simulink model "feng_ct"  (R2016b)
settings: Solver=VariableStepAuto  StartTime=0.0  StopTime=5000  RelTol=1e-3  EnableMultiTasking=on
undefined symbols (not defined in the file or in its folder): fft_stages, output_len_bits, xengbits
undefined symbols (not defined in the file): input_bits, total_bits, total_bits2
libraries: xbsIndex_r4 x10571, casper_library_misc x48, casper_library_scopes x9, xps_library x2
(part 26 of 81)

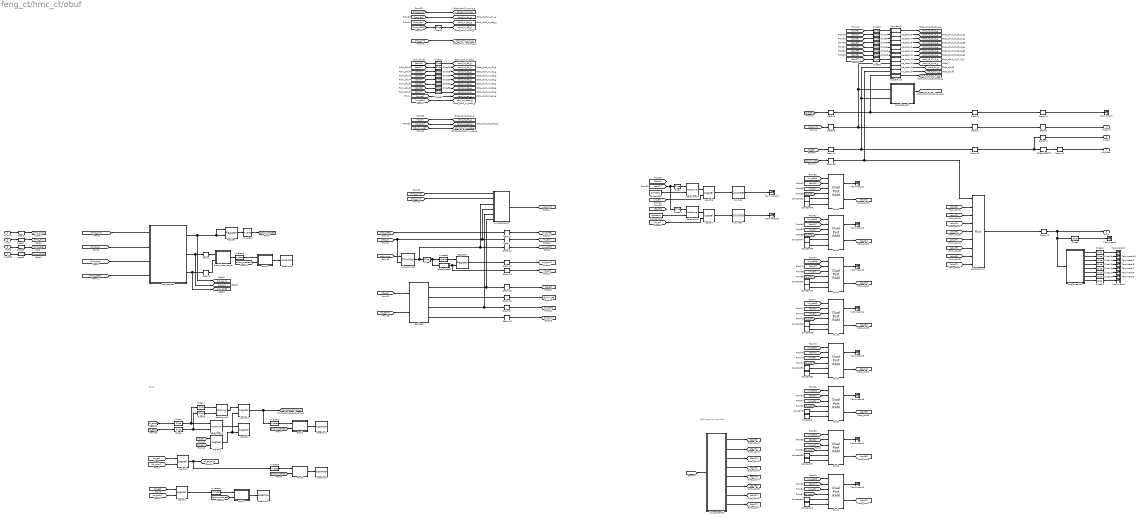
== system feng_ct/hmc_ct/obuf ==
  note: Errors
  note: Eight parallel channels.
  in_sync : Inport
  in_dv : Inport  Port=2
  in_tag : Inport  Port=3
  in_d256 : Inport  Port=4
  Assert : xbsIndex_r4/Assert  assert_type=on  type_source=Explicitly  gui_display_data_type=Boolean  arith_type=Boolean  n_bits=16  bin_pt=14  preci_type=Single  exp_width=8  frac_width=24  assert_rate=on  rate_source=Explicitly  period=1  output_port=on  block_type=assert
  Assert1 : xbsIndex_r4/Assert  assert_type=on  type_source=Explicitly  gui_display_data_type=Boolean  arith_type=Boolean  n_bits=16  bin_pt=14  preci_type=Single  exp_width=8  frac_width=24  assert_rate=on  rate_source=Explicitly  period=1  output_port=on  block_type=assert
  Assert2 : xbsIndex_r4/Assert  assert_type=on  type_source=Explicitly  gui_display_data_type=Fixed-point  arith_type=Unsigned  n_bits=9  bin_pt=0  preci_type=Single  exp_width=8  frac_width=24  assert_rate=on  rate_source=Explicitly  period=1  output_port=on  block_type=assert
  Assert3 : xbsIndex_r4/Assert  assert_type=on  type_source=Explicitly  gui_display_data_type=Fixed-point  arith_type=Unsigned  n_bits=256  bin_pt=0  preci_type=Single  exp_width=8  frac_width=24  assert_rate=on  rate_source=Explicitly  period=1  output_port=on  block_type=assert
  Assertion{1..3,5} (4 alike) : Assertion
  Constant{5,36,38,42,44,46,48,50} (8 alike) : xbsIndex_r4/Constant  const=0  gui_display_data_type=Fixed-point  arith_type=Unsigned  n_bits=256  bin_pt=0  preci_type=Single  exp_width=8  frac_width=24  explicit_period=on  period=1  equ=P=C  opselect=C  inp2=PCIN>>17  opr=+  inp1=P  carry=CIN  dbl_ovrd=off  block_type=constant
  Constant{6,37,41,43,45,47,49,51} (8 alike) : xbsIndex_r4/Constant  const=0  gui_display_data_type=Boolean  arith_type=Boolean  n_bits=256  bin_pt=0  preci_type=Single  exp_width=8  frac_width=24  explicit_period=on  period=1  equ=P=C  opselect=C  inp2=PCIN>>17  opr=+  inp1=P  carry=CIN  dbl_ovrd=off  block_type=constant
  Constant52 : xbsIndex_r4/Constant  const=14695  gui_display_data_type=Fixed-point  arith_type=Unsigned  n_bits=fft_stages-1  bin_pt=0  preci_type=Single  exp_width=8  frac_width=24  explicit_period=on  period=1  equ=P=C  opselect=C  inp2=PCIN>>17  opr=+  inp1=P  carry=CIN  dbl_ovrd=off  block_type=constant
  Constant53 : xbsIndex_r4/Constant  const=29031  gui_display_data_type=Fixed-point  arith_type=Unsigned  n_bits=fft_stages-1  bin_pt=0  preci_type=Single  exp_width=8  frac_width=24  explicit_period=on  period=1  equ=P=C  opselect=C  inp2=PCIN>>17  opr=+  inp1=P  carry=CIN  dbl_ovrd=off  block_type=constant
  Counter : xbsIndex_r4/Counter  cnt_type=Free Running  cnt_to=Inf  operation=Up  start_count=0  cnt_by_val=1  arith_type=Unsigned  n_bits=32  bin_pt=0  load_pin=off  rst=off  en=on  explicit_period=on  period=1  use_behavioral_HDL=off  implementation=Fabric  dbl_ovrd=off  block_type=counter
  Counter1 : xbsIndex_r4/Counter  cnt_type=Free Running  cnt_to=Inf  operation=Up  start_count=0  cnt_by_val=1  arith_type=Unsigned  n_bits=32  bin_pt=0  load_pin=off  rst=off  en=on  explicit_period=on  period=1  use_behavioral_HDL=off  implementation=Fabric  dbl_ovrd=off  block_type=counter
  Delay1 : xbsIndex_r4/Delay  rst=off  infoeditControl=Selection of Reset will increase slice count due to use of real FFs and instead of SRLs  en=off  latency=1  reg_retiming=off  dbl_ovrd=off  block_type=delay
      settings: infoedit=Hardware notes: A delay line is a chain, each link of which is an SRL16 or SRL32 followed by a flip-flop.
  Delay{4,7,10,12..18} (10 alike) : xbsIndex_r4/Delay  rst=off  infoeditControl=Selection of Reset will increase slice count due to use of real FFs and instead of SRLs  en=off  latency=2  reg_retiming=off  dbl_ovrd=off  block_type=delay
      settings: infoedit=Hardware notes: A delay line is a chain, each link of which is an SRL16 or SRL32 followed by a flip-flop.
  Delay{3,11,37,45} (4 alike) : xbsIndex_r4/Delay  rst=off  infoeditControl=Selection of Reset will increase slice count due to use of real FFs and instead of SRLs  en=off  latency=3  reg_retiming=off  dbl_ovrd=off  block_type=delay
      settings: infoedit=Hardware notes: A delay line is a chain, each link of which is an SRL16 or SRL32 followed by a flip-flop.
  Delay2 : xbsIndex_r4/Delay  rst=off  infoeditControl=Selection of Reset will increase slice count due to use of real FFs and instead of SRLs  en=off  latency=1  reg_retiming=off  dbl_ovrd=off  block_type=delay
      settings: infoedit=Hardware notes: A delay line is a chain, each link of which is an SRL16 or SRL32 followed by a flip-flop.
  Delay{6,8,36,42} (4 alike) : xbsIndex_r4/Delay  rst=off  infoeditControl=Selection of Reset will increase slice count due to use of real FFs and instead of SRLs  en=off  latency=pkt_buffer_latency  reg_retiming=off  dbl_ovrd=off  block_type=delay
      settings: infoedit=Hardware notes: A delay line is a chain, each link of which is an SRL16 or SRL32 followed by a flip-flop.
  Delay43 : xbsIndex_r4/Delay  rst=off  infoeditControl=Selection of Reset will increase slice count due to use of real FFs and instead of SRLs  en=off  latency=omux_latency  reg_retiming=off  dbl_ovrd=off  block_type=delay
      settings: infoedit=Hardware notes: A delay line is a chain, each link of which is an SRL16 or SRL32 followed by a flip-flop.
  Delay5 : xbsIndex_r4/Delay  rst=off  infoeditControl=Selection of Reset will increase slice count due to use of real FFs and instead of SRLs  en=off  latency=omux_latency  reg_retiming=off  dbl_ovrd=off  block_type=delay
      settings: infoedit=Hardware notes: A delay line is a chain, each link of which is an SRL16 or SRL32 followed by a flip-flop.
  Delay9 : xbsIndex_r4/Delay  rst=off  infoeditControl=Selection of Reset will increase slice count due to use of real FFs and instead of SRLs  en=off  latency=omux_latency  reg_retiming=off  dbl_ovrd=off  block_type=delay
      settings: infoedit=Hardware notes: A delay line is a chain, each link of which is an SRL16 or SRL32 followed by a flip-flop.
  Inverter{1..6} (6 alike) : xbsIndex_r4/Inverter  en=off  latency=0  dbl_ovrd=off  block_type=inv
  Logical1 : xbsIndex_r4/Logical  logical_function=AND  inputs=2  en=off  latency=1  precision=Full  arith_type=Unsigned  n_bits=16  bin_pt=0  align_bp=on  dbl_ovrd=off  block_type=logical
  Logical{2..3,6..7,9} (5 alike) : xbsIndex_r4/Logical  logical_function=AND  inputs=2  en=off  latency=0  precision=Full  arith_type=Unsigned  n_bits=16  bin_pt=0  align_bp=on  dbl_ovrd=off  block_type=logical
  Logical4 : xbsIndex_r4/Logical  logical_function=AND  inputs=2  en=off  latency=1  precision=Full  arith_type=Unsigned  n_bits=16  bin_pt=0  align_bp=on  dbl_ovrd=off  block_type=logical
  Register : xbsIndex_r4/Register  init=0  rst=off  en=on  dbl_ovrd=off  block_type=register
  Register1 : xbsIndex_r4/Register  init=0  rst=off  en=on  dbl_ovrd=off  block_type=register
  Relational{2..4,6} (4 alike) : xbsIndex_r4/Relational  mode=a=b  op_type=Bool  en=off  latency=0  dbl_ovrd=off  block_type=relational
  Slice : xbsIndex_r4/Slice  nbits=1  boolean_output=on  mode=Upper Bit Location + Width  bit1=0  base1=MSB of Input  bit0=0  base0=LSB of Input  dbl_ovrd=off  block_type=slice
  Slice1 : xbsIndex_r4/Slice  nbits=1  boolean_output=off  mode=Two Bit Locations  bit1=0  base1=MSB of Input  bit0=0  base0=LSB of Input  dbl_ovrd=off  block_type=slice
  Slice{10..16,20} (8 alike) : xbsIndex_r4/Slice  nbits=9  boolean_output=off  mode=Lower Bit Location + Width  bit1=0  base1=MSB of Input  bit0=0  base0=LSB of Input  dbl_ovrd=off  block_type=slice
  Slice17 : xbsIndex_r4/Slice  nbits=1  boolean_output=off  mode=Two Bit Locations  bit1=0  base1=MSB of Input  bit0=5  base0=LSB of Input  dbl_ovrd=off  block_type=slice
  Slice18 : xbsIndex_r4/Slice  nbits=1  boolean_output=off  mode=Two Bit Locations  bit1=0  base1=MSB of Input  bit0=5  base0=LSB of Input  dbl_ovrd=off  block_type=slice
  Slice19 : xbsIndex_r4/Slice  nbits=15  boolean_output=off  mode=Upper Bit Location + Width  bit1=-1  base1=MSB of Input  bit0=0  base0=LSB of Input  dbl_ovrd=off  block_type=slice
  Slice{6..9,22..34} (17 alike) : xbsIndex_r4/Slice  nbits=fft_stages-1  boolean_output=off  mode=Upper Bit Location + Width  bit1=-1*(16-(fft_stages-1))  base1=MSB of Input  bit0=0  base0=LSB of Input  dbl_ovrd=off  block_type=slice
  Slice3 : xbsIndex_r4/Slice  nbits=15  boolean_output=off  mode=Upper Bit Location + Width  bit1=-1  base1=MSB of Input  bit0=0  base0=LSB of Input  dbl_ovrd=off  block_type=slice
  Slice4 : xbsIndex_r4/Slice  nbits=16  boolean_output=off  mode=Upper Bit Location + Width  bit1=0  base1=MSB of Input  bit0=0  base0=LSB of Input  dbl_ovrd=off  block_type=slice
  Slice5 : xbsIndex_r4/Slice  nbits=1  boolean_output=off  mode=Two Bit Locations  bit1=0  base1=MSB of Input  bit0=3  base0=LSB of Input  dbl_ovrd=off  block_type=slice
  Terminator{1,3..19,22..23} (20 alike) : Terminator
  bus_expand1 : Subsystem  AncestorBlock=casper_library_flow_control/bus_expand  mask(bus_expand){mode=divisions of equal size, outputNum=8, outputWidth=32, outputBinaryPt=0, outputArithmeticType=0, show_format=on, outputToWorkspace=off, variablePrefix=out, outputToModelAsWell=on}
      mask prompts: outputNum "Number of outputs:"; outputWidth "Output width:"; outputBinaryPt "Output binary point position:"; outputArithmeticType "Output arithmetic type (ufix=0, fix=1, bool=2):"; show_format "Print format string?"; outputToWorkspace "Output to workspace?"; variablePrefix "Variable name prefix:"; outputToModelAsWell "Output to model as well?"
      mask help:
      | Expands a 'bus' made using a bus_create or Xilinx
      | concat block.
      | The input will be divided into the specified number
      | of outputs with the specified arithmetic types.
      | Divisions are made from most significant bit.
      mask init: same as feng_ct/bus_expand1
      settings: AttributesFormatString=8 outputs: uf32.0,uf32.0,uf32.0,uf32.0,uf32.0,uf32.0,uf32.0,uf32.0,
      mask TypeOptions mode: divisions of equal size | divisions of arbitrary size
      mask Callback mode: bus_expand_callback();
      mask Callback outputWidth: bus_expand_callback();
      mask Callback outputToWorkspace: bus_expand_callback();
  bus_expand3 : Subsystem  AncestorBlock=casper_library_flow_control/bus_expand  mask(bus_expand){mode=divisions of equal size, outputNum=8, outputWidth=32, outputBinaryPt=0, outputArithmeticType=0, show_format=off, outputToWorkspace=off, variablePrefix=out, outputToModelAsWell=on}
      mask prompts: outputNum "Number of outputs:"; outputWidth "Output width:"; outputBinaryPt "Output binary point position:"; outputArithmeticType "Output arithmetic type (ufix=0, fix=1, bool=2):"; show_format "Print format string?"; outputToWorkspace "Output to workspace?"; variablePrefix "Variable name prefix:"; outputToModelAsWell "Output to model as well?"
      mask help:
      | Expands a 'bus' made using a bus_create or Xilinx
      | concat block.
      | The input will be divided into the specified number
      | of outputs with the specified arithmetic types.
      | Divisions are made from most significant bit.
      mask init: same as feng_ct/bus_expand1
      settings: AttributesFormatString=8 outputs
      mask TypeOptions mode: divisions of equal size | divisions of arbitrary size
      mask Callback mode: bus_expand_callback();
      mask Callback outputWidth: bus_expand_callback();
      mask Callback outputToWorkspace: bus_expand_callback();
  check_data_length : Subsystem
  edge_detect : Subsystem  AncestorBlock=casper_library_misc/edge_detect  mask(edge_detect){edge=Both, polarity=Active High, x_in=[0 0.08 0.08 0.16 0.16 0.24 0.24 0.32 0.32 0.4], y_in=[-1 -1  1  1  1  1  1  1  1  1], x_out=[0.6 0.68 0.68 0.76 0.76 0.84 0.84 0.92 0.92 1], y_out=[-1 -1  1  1 -1 -1 -1 -1 -1 -1]}
      mask prompts: edge "Edge Type"; polarity "Output Polarity"; x_in "Input X Positions"; y_in "Input Y Positions"; x_out "Output X Positions"; y_out "Output Y Positions"
      mask help: Output is active for one-cycle after each edge of the specified type (i.e. rising, falling or both).
      mask init: same as feng_ct/edge_detect1
      settings: AttributesFormatString=|
      | both edges
      | active high
      mask Help: Output is active for one-cycle after each edge of the specified type (i.e. rising, falling, or both).  Latency is zero.
      mask TypeOptions edge: Rising | Falling | Both
      mask TypeOptions polarity: Active High | Active Low
      mask Display:
      | plot(x_in_num,0.5+y_in_num*0.2);
      | plot(x_out_num,0.5+y_out_num*0.2);
  edge_detect1 : casper_library_misc/edge_detect  edge=Rising  polarity=Active High  x_in=[0 0.08 0.08 0.16 0.16 0.24 0.24 0.32 0.32 0.4]  y_in="[-1 -1  1  1  1  1  1  1  1  1]"  x_out=[0.6 0.68 0.68 0.76 0.76 0.84 0.84 0.92 0.92 1]  y_out="[-1 -1  1  1 -1 -1 -1 -1 -1 -1]"
  error1 : Subsystem
  error2 : Subsystem
  error3 : Subsystem
  error4 : Subsystem
  gen_freq_calc : Subsystem  mask{pkt_len_bits=5, lat=3}
      mask prompts: pkt_len_bits "Packet length bits"; lat "Latency"
      mask init:
      | display_string = sprintf('latency=%i', 7 * lat);
      | set_param(gcb, 'AttributesFormatString', display_string);
      settings: AttributesFormatString=latency=21
  obuf0 : xbsIndex_r4/Dual Port RAM  depth=2^(output_len_bits + 2)  initVector=ones(1, 2^(output_len_bits + 2))  distributed_mem=Block RAM  init_a=0  init_b=0  rst_a=off  rst_b=off  en_a=off  en_b=off  latency=pkt_buffer_latency  write_mode_A=Read Before Write  write_mode_B=Read Before Write  optimize=Area  dbl_ovrd=off  block_type=dpram
  obuf{1..7} (7 alike) : xbsIndex_r4/Dual Port RAM  depth=2^(output_len_bits + 2)  initVector=zeros(1, 2^(output_len_bits + 2))  distributed_mem=Block RAM  init_a=0  init_b=0  rst_a=off  rst_b=off  en_a=off  en_b=off  latency=pkt_buffer_latency  write_mode_A=Read Before Write  write_mode_B=Read Before Write  optimize=Area  dbl_ovrd=off  block_type=dpram
  pkt_data_mux : xbsIndex_r4/Mux  inputs=8  en=off  latency=omux_latency  precision=Full  arith_type=Unsigned  n_bits=16  bin_pt=14  quantization=Truncate  overflow=Wrap  dbl_ovrd=off  block_type=mux
  read_gen : Subsystem
  sync_generator : Subsystem
  tag_reorder : Subsystem
  we_delay1 : Subsystem  AncestorBlock=casper_library_delays/pipeline  mask(pipeline){latency=21}
      mask help:
      | An explicitly laid-out delay line to avoid mapping to SRL16s
      | for use in pipelining to help achieve timing closure.
      mask init:
      | pipeline_init(gcb,'latency',latency);
      settings: AttributesFormatString=Latency = %<latency>
      mask Display:
      | port_label('input', 1, 'd');
      | port_label('output', 1, 'q');
      | disp(['Z^-', num2str(latency)]);
  we_delay10 : Subsystem  AncestorBlock=casper_library_delays/pipeline  mask(pipeline){latency=21}
      mask help:
      | An explicitly laid-out delay line to avoid mapping to SRL16s
      | for use in pipelining to help achieve timing closure.
      mask init:
      | pipeline_init(gcb,'latency',latency);
      settings: AttributesFormatString=Latency = %<latency>
      mask Display:
      | port_label('input', 1, 'd');
      | port_label('output', 1, 'q');
      | disp(['Z^-', num2str(latency)]);
  we_delay11 : Subsystem  AncestorBlock=casper_library_delays/pipeline  mask(pipeline){latency=21}
      mask help:
      | An explicitly laid-out delay line to avoid mapping to SRL16s
      | for use in pipelining to help achieve timing closure.
      mask init:
      | pipeline_init(gcb,'latency',latency);
      settings: AttributesFormatString=Latency = %<latency>
      mask Display:
      | port_label('input', 1, 'd');
      | port_label('output', 1, 'q');
      | disp(['Z^-', num2str(latency)]);
  we_delay12 : Subsystem  AncestorBlock=casper_library_delays/pipeline  mask(pipeline){latency=21}
      mask help:
      | An explicitly laid-out delay line to avoid mapping to SRL16s
      | for use in pipelining to help achieve timing closure.
      mask init:
      | pipeline_init(gcb,'latency',latency);
      settings: AttributesFormatString=Latency = %<latency>
      mask Display:
      | port_label('input', 1, 'd');
      | port_label('output', 1, 'q');
      | disp(['Z^-', num2str(latency)]);
  we_delay13 : Subsystem  AncestorBlock=casper_library_delays/pipeline  mask(pipeline){latency=21}
      mask help:
      | An explicitly laid-out delay line to avoid mapping to SRL16s
      | for use in pipelining to help achieve timing closure.
      mask init:
      | pipeline_init(gcb,'latency',latency);
      settings: AttributesFormatString=Latency = %<latency>
      mask Display:
      | port_label('input', 1, 'd');
      | port_label('output', 1, 'q');
      | disp(['Z^-', num2str(latency)]);
  we_delay2 : Subsystem  AncestorBlock=casper_library_delays/pipeline  mask(pipeline){latency=21}
      mask help:
      | An explicitly laid-out delay line to avoid mapping to SRL16s
      | for use in pipelining to help achieve timing closure.
      mask init:
      | pipeline_init(gcb,'latency',latency);
      settings: AttributesFormatString=Latency = %<latency>
      mask Display:
      | port_label('input', 1, 'd');
      | port_label('output', 1, 'q');
      | disp(['Z^-', num2str(latency)]);
  we_delay3 : Subsystem  AncestorBlock=casper_library_delays/pipeline  mask(pipeline){latency=21}
      mask help:
      | An explicitly laid-out delay line to avoid mapping to SRL16s
      | for use in pipelining to help achieve timing closure.
      mask init:
      | pipeline_init(gcb,'latency',latency);
      settings: AttributesFormatString=Latency = %<latency>
      mask Display:
      | port_label('input', 1, 'd');
      | port_label('output', 1, 'q');
      | disp(['Z^-', num2str(latency)]);
  we_delay5 : Subsystem  AncestorBlock=casper_library_delays/pipeline  mask(pipeline){latency=21}
      mask help:
      | An explicitly laid-out delay line to avoid mapping to SRL16s
      | for use in pipelining to help achieve timing closure.
      mask init:
      | pipeline_init(gcb,'latency',latency);
      settings: AttributesFormatString=Latency = %<latency>
      mask Display:
      | port_label('input', 1, 'd');
      | port_label('output', 1, 'q');
      | disp(['Z^-', num2str(latency)]);
  we_delay6 : Subsystem  AncestorBlock=casper_library_delays/pipeline  mask(pipeline){latency=21}
      mask help:
      | An explicitly laid-out delay line to avoid mapping to SRL16s
      | for use in pipelining to help achieve timing closure.
      mask init:
      | pipeline_init(gcb,'latency',latency);
      settings: AttributesFormatString=Latency = %<latency>
      mask Display:
      | port_label('input', 1, 'd');
      | port_label('output', 1, 'q');
      | disp(['Z^-', num2str(latency)]);
  we_delay7 : Subsystem  AncestorBlock=casper_library_delays/pipeline  mask(pipeline){latency=21}
      mask help:
      | An explicitly laid-out delay line to avoid mapping to SRL16s
      | for use in pipelining to help achieve timing closure.
      mask init:
      | pipeline_init(gcb,'latency',latency);
      settings: AttributesFormatString=Latency = %<latency>
      mask Display:
      | port_label('input', 1, 'd');
      | port_label('output', 1, 'q');
      | disp(['Z^-', num2str(latency)]);
  we_delay8 : Subsystem  AncestorBlock=casper_library_delays/pipeline  mask(pipeline){latency=21}
      mask help:
      | An explicitly laid-out delay line to avoid mapping to SRL16s
      | for use in pipelining to help achieve timing closure.
      mask init:
      | pipeline_init(gcb,'latency',latency);
      settings: AttributesFormatString=Latency = %<latency>
      mask Display:
      | port_label('input', 1, 'd');
      | port_label('output', 1, 'q');
      | disp(['Z^-', num2str(latency)]);
  we_delay9 : Subsystem  AncestorBlock=casper_library_delays/pipeline  mask(pipeline){latency=21}
      mask help:
      | An explicitly laid-out delay line to avoid mapping to SRL16s
      | for use in pipelining to help achieve timing closure.
      mask init:
      | pipeline_init(gcb,'latency',latency);
      settings: AttributesFormatString=Latency = %<latency>
      mask Display:
      | port_label('input', 1, 'd');
      | port_label('output', 1, 'q');
      | disp(['Z^-', num2str(latency)]);
  write_counter : xbsIndex_r4/Counter  cnt_type=Free Running  cnt_to=Inf  operation=Up  start_count=0  cnt_by_val=1  arith_type=Unsigned  n_bits=10  bin_pt=0  load_pin=off  rst=on  en=on  explicit_period=on  period=1  use_behavioral_HDL=off  implementation=Fabric  dbl_ovrd=off  block_type=counter
  out_sync : Outport
  out_dv : Outport  Port=2
  out_d : Outport  Port=3
  pkt_start : Outport  Port=4
  tag scope: obuf_ct_addr_err_g=global, obuf_dv_g=global, obuf_in_d0_g=global, obuf_in_dv_g=global, obuf_in_sync_g=global, obuf_in_tag_g=global, obuf_mux_g=global, obuf_premux_freq_ctr_g=global, obuf_proc_sync_g=global, obuf_rd_addr_g=global, obuf_rd_addr_out_g=global, obuf_rd_d0_0_g=global, obuf_rd_d1_0_g=global, obuf_rd_d2_0_g=global, obuf_rd_d3_0_g=global, obuf_rd_d4_0_g=global, obuf_rd_d5_0_g=global, obuf_rd_d6_0_g=global, obuf_rd_d7_0_g=global, obuf_rd_en_g=global, obuf_rd_mux_sel_g=global, obuf_rd_sync_g=global, obuf_wr_addr_g=global, obuf_wr_d0_g=global, obuf_wr_d1_g=global, obuf_wr_d2_g=global, obuf_wr_d3_g=global, obuf_wr_d4_g=global, obuf_wr_d5_g=global, obuf_wr_d6_g=global, obuf_wr_d7_g=global, obuf_wr_en_g=global, proc_d256=global, proc_dv=global, proc_sync=global, rd_go_err_g=global
  wires:
  in_dv/1 -> Assert1/1  "IN_dv"
  in_tag/1 -> Assert2/1
  in_sync/1 -> Assert/1  "IN_sync"
  [rd_en] -> Logical9/1
  [wr_en] -> Logical9/2
  Logical9/1 -> Logical3/2, Logical2/2
  [rd_go] -> Logical4/1
  [rd_busy] -> Logical4/2
  Logical4/1 -> Inverter5/1, [rd_go_err_g]  "GO_ERROR"
  in_d256/1 -> Assert3/1
  [wr_addr] -> Slice5/1
  [rd_addr] -> Slice1/1
  Slice5/1 -> Slice17/1, Relational2/1  "WR_ADDR7"
  Slice1/1 -> Slice18/1, Relational2/2  "RD_ADDR7"
  Relational2/1 -> Logical2/1
  Logical3/1 -> Inverter2/1, [obuf_ct_addr_err_g]  "BANK_CLASH"
  Slice18/1 -> Relational3/2  "RD_ADDR2"
  Slice17/1 -> Relational3/1  "WR_ADDR2"
  Relational3/1 -> Logical3/1
  [hmc_d256] -> tag_reorder/4(in_d256)
  [hmc_tag] -> tag_reorder/3(in_tag)
  [hmc_dv] -> tag_reorder/2(in_dv)
  [hmc_sync] -> tag_reorder/1(in_sync)
  check_data_length/1(error) -> Inverter6/1
  tag_reorder/3(out_d256) -> [proc_d256], Delay2/1
  tag_reorder/2(out_dv) -> [proc_dv], Delay1/1
  Inverter6/1 -> error4/1(err)
  error4/1(err_out) -> Assertion5/1
  tag_reorder/1(out_sync) -> [proc_sync], Register/2, Register/1  "PROC_sync"
  Register/1 -> Inverter1/1
  Inverter1/1 -> [errors_masked]
  [errors_masked] -> error4/2(armed)
  Delay1/1 -> check_data_length/1(dv)
  Delay2/1 -> check_data_length/2(data)
  [rd_go] -> Logical1/1
  [rd_busy] -> Logical1/2
  Logical1/1 -> Inverter4/1  "RD_BUSY_CLASH"
  Inverter4/1 -> error2/1(err)
  error2/1(err_out) -> Assertion2/1
  [errors_masked] -> error2/2(armed)
  [wr_en] -> [obuf_wr_en_g]
  [wr_addr] -> [obuf_wr_addr_g]
  [rd_addr] -> [obuf_rd_addr_g]
  [rd_mux_sel] -> [obuf_rd_mux_sel_g]
  [rd_en] -> [obuf_rd_en_g]
  [hmc_sync] -> [obuf_in_sync_g]
  [hmc_d256] -> Slice22/1
  Slice22/1 -> [obuf_in_d0_g]
  [hmc_dv] -> [obuf_in_dv_g]
  [hmc_tag] -> [obuf_in_tag_g]
  [dbuf0] -> Slice27/1
  Slice27/1 -> [obuf_wr_d0_g]
  [dbuf1] -> Slice28/1
  [dbuf2] -> Slice29/1
  [dbuf3] -> Slice30/1
  [dbuf4] -> Slice31/1
  [dbuf5] -> Slice32/1
  [dbuf6] -> Slice33/1
  [dbuf7] -> Slice34/1
  Slice28/1 -> [obuf_wr_d1_g]
  Slice29/1 -> [obuf_wr_d2_g]
  Slice30/1 -> [obuf_wr_d3_g]
  Slice31/1 -> [obuf_wr_d4_g]
  Slice32/1 -> [obuf_wr_d5_g]
  Slice33/1 -> [obuf_wr_d6_g]
  Slice34/1 -> [obuf_wr_d7_g]
  [dbuf5] -> obuf5/2
  [wr_addr] -> obuf5/1
  [wr_en] -> obuf5/3
  [rd_addr] -> obuf5/4
  Constant5/1 -> obuf5/5
  Constant6/1 -> obuf5/6
  bus_expand1/8(lsb_out1) -> Slice20/1
  bus_expand1/7(out2) -> Slice10/1
  bus_expand1/6(out3) -> Slice11/1
  bus_expand1/5(out4) -> Slice12/1
  Slice12/1 -> Terminator7/1  "tag3"
  Slice11/1 -> Terminator6/1  "tag2"
  Slice10/1 -> Terminator5/1  "tag1"
  Slice20/1 -> Terminator4/1  "tag0"
  bus_expand1/1(msb_out8) -> Slice16/1
  bus_expand1/2(out7) -> Slice15/1
  bus_expand1/3(out6) -> Slice14/1
  Slice16/1 -> Terminator17/1
  Slice15/1 -> Terminator16/1
  Slice14/1 -> Terminator9/1
  Slice13/1 -> Terminator8/1
  bus_expand1/4(out5) -> Slice13/1
  obuf5/2 -> [obuf5]
  obuf5/1 -> Terminator18/1
  [dbuf6] -> obuf6/2
  [wr_addr] -> obuf6/1
  [wr_en] -> obuf6/3
  [rd_addr] -> obuf6/4
  Constant36/1 -> obuf6/5
  Constant37/1 -> obuf6/6
  obuf6/2 -> [obuf6]
  obuf6/1 -> Terminator19/1
  [dbuf7] -> obuf7/2
  [wr_addr] -> obuf7/1
  [wr_en] -> obuf7/3
  [rd_addr] -> obuf7/4
  Constant38/1 -> obuf7/5
  Constant41/1 -> obuf7/6
  obuf7/2 -> [obuf7]
  obuf7/1 -> Terminator10/1
  [dbuf0] -> obuf0/2
  [wr_addr] -> obuf0/1
  [wr_en] -> obuf0/3
  [rd_addr] -> obuf0/4
  Constant42/1 -> obuf0/5
  Constant43/1 -> obuf0/6
  obuf0/2 -> [obuf0]
  obuf0/1 -> Terminator11/1
  [dbuf1] -> obuf1/2
  [wr_addr] -> obuf1/1
  [wr_en] -> obuf1/3
  [rd_addr] -> obuf1/4
  Constant44/1 -> obuf1/5
  Constant45/1 -> obuf1/6
  obuf1/2 -> [obuf1]
  obuf1/1 -> Terminator12/1
  [dbuf2] -> obuf2/2
  [wr_addr] -> obuf2/1
  [wr_en] -> obuf2/3
  [rd_addr] -> obuf2/4
  Constant46/1 -> obuf2/5
  Constant47/1 -> obuf2/6
  obuf2/2 -> [obuf2]
  obuf2/1 -> Terminator13/1
  [dbuf3] -> obuf3/2
  [wr_addr] -> obuf3/1
  [wr_en] -> obuf3/3
  [rd_addr] -> obuf3/4
  Constant48/1 -> obuf3/5
  Constant49/1 -> obuf3/6
  obuf3/2 -> [obuf3]
  obuf3/1 -> Terminator14/1
  [dbuf4] -> obuf4/2
  [wr_addr] -> obuf4/1
  [wr_en] -> obuf4/3
  [rd_addr] -> obuf4/4
  Constant50/1 -> obuf4/5
  Constant51/1 -> obuf4/6
  obuf4/2 -> [obuf4]
  obuf4/1 -> Terminator15/1
  [rd_mux_sel] -> Delay36/1
  [obuf4] -> pkt_data_mux/6
  [obuf6] -> pkt_data_mux/8
  [obuf5] -> pkt_data_mux/7
  [obuf7] -> pkt_data_mux/9
  [obuf3] -> pkt_data_mux/5
  [obuf2] -> pkt_data_mux/4
  [obuf0] -> pkt_data_mux/2
  [obuf1] -> pkt_data_mux/3
  [rd_en] -> Delay42/1
  Delay45/1 -> out_d/1, Slice4/1, bus_expand1/1(bus_in)
  Delay37/1 -> out_dv/1  "out_dv"
  pkt_data_mux/1 -> Delay45/1
  [wr_d256] -> bus_expand3/1(bus_in)
  bus_expand3/1(msb_out8) -> [dbuf0]
  bus_expand3/2(out7) -> [dbuf1]
  bus_expand3/3(out6) -> [dbuf2]
  bus_expand3/4(out5) -> [dbuf3]
  bus_expand3/5(out4) -> [dbuf4]
  bus_expand3/6(out3) -> [dbuf5]
  bus_expand3/7(out2) -> [dbuf6]  "DATA_TAG"
  bus_expand3/8(lsb_out1) -> [dbuf7]
  Slice4/1 -> Terminator3/1  "out_freq"
  Delay36/1 -> pkt_data_mux/1, we_delay3/1(d)  "obuf_mux"
  Delay42/1 -> gen_freq_calc/2(dv), we_delay2/1(d), Delay43/1  "obuf_en"
  [obuf0] -> Slice23/1
  Slice23/1 -> we_delay5/1(d)  "obuf0"
  [obuf7] -> Slice26/1
  Slice26/1 -> we_delay12/1(d)
  [obuf1] -> Slice7/1
  Slice7/1 -> we_delay6/1(d)
  [obuf2] -> Slice8/1
  Slice8/1 -> we_delay7/1(d)
  [obuf3] -> Slice9/1
  Slice9/1 -> we_delay8/1(d)
  [obuf4] -> Slice6/1
  Slice6/1 -> we_delay9/1(d)
  [obuf5] -> Slice24/1
  Slice24/1 -> we_delay10/1(d)
  [obuf6] -> Slice25/1
  Slice25/1 -> we_delay11/1(d)
  we_delay2/1(q) -> [obuf_dv_g]
  we_delay3/1(q) -> [obuf_mux_g]
  we_delay13/1(q) -> [obuf_rd_addr_out_g]
  we_delay5/1(q) -> [obuf_rd_d0_0_g]
  we_delay6/1(q) -> [obuf_rd_d1_0_g]
  we_delay8/1(q) -> [obuf_rd_d3_0_g]
  we_delay7/1(q) -> [obuf_rd_d2_0_g]
  we_delay12/1(q) -> [obuf_rd_d7_0_g]
  we_delay11/1(q) -> [obuf_rd_d6_0_g]
  we_delay9/1(q) -> [obuf_rd_d4_0_g]
  we_delay10/1(q) -> [obuf_rd_d5_0_g]
  Delay5/1 -> Delay3/1  "out_sync"
  [rd_addr] -> Delay8/1
  Delay8/1 -> we_delay13/1(d), Delay9/1
  Delay11/1 -> Terminator1/1  "out_addr"
  Delay9/1 -> Delay11/1
  edge_detect1/1 -> Delay10/1
  Delay43/1 -> Delay37/1, edge_detect1/1
  Delay10/1 -> pkt_start/1  "out_pkt_start"
  we_delay1/1(q) -> [obuf_rd_sync_g]
  Delay6/1 -> gen_freq_calc/1(sync), we_delay1/1(d), Delay5/1
  [dbuf7] -> Slice19/1, Slice3/1
  Constant52/1 -> Relational4/2
  Relational4/1 -> Logical6/1
  [wr_en] -> Logical6/2
  Logical6/1 -> Counter/1  "WR_14695"
  Counter/1 -> Terminator22/1  "20504"
  Constant53/1 -> Relational6/2
  Relational6/1 -> Logical7/1
  [wr_en] -> Logical7/2
  Logical7/1 -> Counter1/1  "WR_29031"
  Counter1/1 -> Terminator23/1  "22552"
  Slice3/1 -> Relational4/1
  Slice19/1 -> Relational6/1
  Assert/1 -> [hmc_sync]
  Assert1/1 -> [hmc_dv]
  Assert2/1 -> [hmc_tag]
  Assert3/1 -> [hmc_d256]
  Inverter2/1 -> error1/1(err)
  error1/1(err_out) -> Assertion1/1
  [errors_masked] -> error1/2(armed)
  Inverter5/1 -> error3/1(err)
  error3/1(err_out) -> Assertion3/1
  [errors_masked] -> error3/2(armed)
  Delay3/1 -> out_sync/1
  gen_freq_calc/2(freq) -> [obuf_premux_freq_ctr_g]
  [proc_sync] -> write_counter/1
  [proc_dv] -> write_counter/2, sync_generator/4(wr_en), Delay7/1
  write_counter/1 -> sync_generator/3(wr_addr), Delay12/1, Slice/1  "WR_addr"
  Slice/1 -> Inverter3/1, edge_detect/1(in)  "WR_bank"
  Inverter3/1 -> Register1/1
  edge_detect/1(out) -> Delay14/1, Register1/2  "RD_go"
  Register1/1 -> Delay13/1
  read_gen/2(mux_sel) -> Delay16/1
  read_gen/1(dv) -> sync_generator/6(rd_en), Delay15/1
  read_gen/3(addr) -> Delay17/1, sync_generator/5(rd_addr)
  read_gen/4(rd_busy) -> Delay18/1
  [rd_bank] -> read_gen/2(bank)
  [rd_go] -> read_gen/1(go)
  [proc_d256] -> Delay4/1
  [proc_sync] -> sync_generator/2(proc_sync)  "PROC_sync"
  [hmc_sync] -> sync_generator/1(hmc_sync)  "HMC_sync"
  Delay4/1 -> [wr_d256]  "WR_d256"
  Delay7/1 -> [wr_en]  "WR_en"
  Delay12/1 -> [wr_addr]  "WR_addr"
  Delay13/1 -> [rd_bank]  "RD_bank"
  Delay14/1 -> [rd_go]  "RD_go"
  Delay15/1 -> [rd_en]  "RD_en"
  Delay16/1 -> [rd_mux_sel]  "RD_muxsel"
  Delay17/1 -> [rd_addr]  "RD_addr"
  Delay18/1 -> [rd_busy]  "RD_busy"
  sync_generator/1(sync) -> [rd_sync]  "RD_sync"
  [rd_sync] -> Delay6/1
  [proc_sync] -> [obuf_proc_sync_g]

== system feng_ct/hmc_ct/tvg_data_gen ==
  sync : Inport
  dv : Inport  Port=2
  Assert1 : xbsIndex_r4/Assert  assert_type=on  type_source=Explicitly  gui_display_data_type=Boolean  arith_type=Boolean  n_bits=16  bin_pt=14  preci_type=Single  exp_width=8  frac_width=24  assert_rate=on  rate_source=Explicitly  period=1  output_port=on  block_type=assert
  Assert2 : xbsIndex_r4/Assert  assert_type=on  type_source=Explicitly  gui_display_data_type=Boolean  arith_type=Boolean  n_bits=16  bin_pt=14  preci_type=Single  exp_width=8  frac_width=24  assert_rate=on  rate_source=Explicitly  period=1  output_port=on  block_type=assert
  Concat20 : xbsIndex_r4/Concat  num_inputs=4  dbl_ovrd=off  block_type=concat
  Concat21 : xbsIndex_r4/Concat  num_inputs=2  dbl_ovrd=off  block_type=concat
  Delay33 : xbsIndex_r4/Delay  rst=off  infoeditControl=Selection of Reset will increase slice count due to use of real FFs and instead of SRLs  en=off  latency=4  reg_retiming=off  dbl_ovrd=off  block_type=delay
      settings: infoedit=Hardware notes: A delay line is a chain, each link of which is an SRL16 or SRL32 followed by a flip-flop.
  convert_rd_en{,1..3} (4 alike) : xbsIndex_r4/Convert  gui_display_data_type=Fixed-point  arith_type=Unsigned  n_bits=16  bin_pt=0  float_type=Single  exp_bits=8  fraction_bits=24  quantization=Truncate  overflow=Wrap  en=off  latency=0  pipeline=off  dbl_ovrd=off  block_type=convert
      settings: xl_area=[0, 0, 0, 0, 0, 0, 0]
  p0_0 : xbsIndex_r4/Counter  cnt_type=Free Running  cnt_to=Inf  operation=Up  start_count=0  cnt_by_val=4  arith_type=Unsigned  n_bits=input_len_bits + 2  bin_pt=0  load_pin=off  rst=on  en=on  explicit_period=on  period=1  use_behavioral_HDL=off  implementation=Fabric  dbl_ovrd=off  block_type=counter
  p0_1 : xbsIndex_r4/Counter  cnt_type=Free Running  cnt_to=Inf  operation=Up  start_count=1  cnt_by_val=4  arith_type=Unsigned  n_bits=input_len_bits + 2  bin_pt=0  load_pin=off  rst=on  en=on  explicit_period=on  period=1  use_behavioral_HDL=off  implementation=Fabric  dbl_ovrd=off  block_type=counter
  p0_2 : xbsIndex_r4/Counter  cnt_type=Free Running  cnt_to=Inf  operation=Up  start_count=2  cnt_by_val=4  arith_type=Unsigned  n_bits=input_len_bits + 2  bin_pt=0  load_pin=off  rst=on  en=on  explicit_period=on  period=1  use_behavioral_HDL=off  implementation=Fabric  dbl_ovrd=off  block_type=counter
  p0_3 : xbsIndex_r4/Counter  cnt_type=Free Running  cnt_to=Inf  operation=Up  start_count=3  cnt_by_val=4  arith_type=Unsigned  n_bits=input_len_bits + 2  bin_pt=0  load_pin=off  rst=on  en=on  explicit_period=on  period=1  use_behavioral_HDL=off  implementation=Fabric  dbl_ovrd=off  block_type=counter
  d128 : Outport
  wires:
  Assert1/1 -> p0_0/2, p0_3/2, p0_2/2, p0_1/2
  Assert2/1 -> p0_0/1, p0_3/1, p0_2/1, p0_1/1
  dv/1 -> Assert1/1
  sync/1 -> Assert2/1
  convert_rd_en1/1 -> Concat20/2
  convert_rd_en2/1 -> Concat20/3
  p0_1/1 -> convert_rd_en1/1
  convert_rd_en/1 -> Concat20/1
  convert_rd_en3/1 -> Concat20/4
  Concat21/1 -> Delay33/1
  p0_2/1 -> convert_rd_en2/1
  p0_3/1 -> convert_rd_en3/1
  Concat20/1 -> Concat21/1, Concat21/2
  p0_0/1 -> convert_rd_en/1
  Delay33/1 -> d128/1

== system feng_ct/hmc_ct/tvg_data_gen_oneshot ==
  sync : Inport
  dv : Inport  Port=2
  Assert1 : xbsIndex_r4/Assert  assert_type=on  type_source=Explicitly  gui_display_data_type=Boolean  arith_type=Boolean  n_bits=16  bin_pt=14  preci_type=Single  exp_width=8  frac_width=24  assert_rate=on  rate_source=Explicitly  period=1  output_port=on  block_type=assert
  Assert2 : xbsIndex_r4/Assert  assert_type=on  type_source=Explicitly  gui_display_data_type=Boolean  arith_type=Boolean  n_bits=16  bin_pt=14  preci_type=Single  exp_width=8  frac_width=24  assert_rate=on  rate_source=Explicitly  period=1  output_port=on  block_type=assert
  Concat20 : xbsIndex_r4/Concat  num_inputs=8  dbl_ovrd=off  block_type=concat
  Concat21 : xbsIndex_r4/Concat  num_inputs=2  dbl_ovrd=off  block_type=concat
  Constant10 : xbsIndex_r4/Constant  const=0  gui_display_data_type=Boolean  arith_type=Boolean  n_bits=10  bin_pt=0  preci_type=Single  exp_width=8  frac_width=24  explicit_period=on  period=1  equ=P=C  opselect=C  inp2=PCIN>>17  opr=+  inp1=P  carry=CIN  dbl_ovrd=off  block_type=constant
  Constant11 : xbsIndex_r4/Constant  const=1  gui_display_data_type=Boolean  arith_type=Boolean  n_bits=10  bin_pt=0  preci_type=Single  exp_width=8  frac_width=24  explicit_period=on  period=1  equ=P=C  opselect=C  inp2=PCIN>>17  opr=+  inp1=P  carry=CIN  dbl_ovrd=off  block_type=constant
  Constant2 : xbsIndex_r4/Constant  const=1023  gui_display_data_type=Fixed-point  arith_type=Unsigned  n_bits=10  bin_pt=0  preci_type=Single  exp_width=8  frac_width=24  explicit_period=on  period=1  equ=P=C  opselect=C  inp2=PCIN>>17  opr=+  inp1=P  carry=CIN  dbl_ovrd=off  block_type=constant
  Counter : xbsIndex_r4/Counter  cnt_type=Free Running  cnt_to=Inf  operation=Up  start_count=0  cnt_by_val=1  arith_type=Unsigned  n_bits=10  bin_pt=0  load_pin=off  rst=on  en=on  explicit_period=on  period=1  use_behavioral_HDL=off  implementation=Fabric  dbl_ovrd=off  block_type=counter
  Delay1 : xbsIndex_r4/Delay  rst=off  infoeditControl=Selection of Reset will increase slice count due to use of real FFs and instead of SRLs  en=off  latency=1  reg_retiming=off  dbl_ovrd=off  block_type=delay
      settings: infoedit=Hardware notes: A delay line is a chain, each link of which is an SRL16 or SRL32 followed by a flip-flop.
  Logical : xbsIndex_r4/Logical  logical_function=AND  inputs=2  en=off  latency=1  precision=Full  arith_type=Unsigned  n_bits=16  bin_pt=0  align_bp=on  dbl_ovrd=off  block_type=logical
  Mux2 : xbsIndex_r4/Mux  inputs=2  en=off  latency=2  precision=Full  arith_type=Unsigned  n_bits=16  bin_pt=14  quantization=Truncate  overflow=Wrap  dbl_ovrd=off  block_type=mux
  Register : xbsIndex_r4/Register  init=0  rst=on  en=on  dbl_ovrd=off  block_type=register
  Relational : xbsIndex_r4/Relational  mode=a<=b  op_type=Bool  en=off  latency=1  dbl_ovrd=off  block_type=relational
  convert_rd_en{,1..3} (4 alike) : xbsIndex_r4/Convert  gui_display_data_type=Fixed-point  arith_type=Unsigned  n_bits=15  bin_pt=0  float_type=Single  exp_bits=8  fraction_bits=24  quantization=Truncate  overflow=Wrap  en=off  latency=0  pipeline=off  dbl_ovrd=off  block_type=convert
      settings: xl_area=[0, 0, 0, 0, 0, 0, 0]
  p0_0 : xbsIndex_r4/Counter  cnt_type=Free Running  cnt_to=Inf  operation=Up  start_count=0  cnt_by_val=4  arith_type=Unsigned  n_bits=input_len_bits + 2  bin_pt=0  load_pin=off  rst=on  en=on  explicit_period=on  period=1  use_behavioral_HDL=off  implementation=Fabric  dbl_ovrd=off  block_type=counter
  p0_1 : xbsIndex_r4/Counter  cnt_type=Free Running  cnt_to=Inf  operation=Up  start_count=1  cnt_by_val=4  arith_type=Unsigned  n_bits=input_len_bits + 2  bin_pt=0  load_pin=off  rst=on  en=on  explicit_period=on  period=1  use_behavioral_HDL=off  implementation=Fabric  dbl_ovrd=off  block_type=counter
  p0_2 : xbsIndex_r4/Counter  cnt_type=Free Running  cnt_to=Inf  operation=Up  start_count=2  cnt_by_val=4  arith_type=Unsigned  n_bits=input_len_bits + 2  bin_pt=0  load_pin=off  rst=on  en=on  explicit_period=on  period=1  use_behavioral_HDL=off  implementation=Fabric  dbl_ovrd=off  block_type=counter
  p0_3 : xbsIndex_r4/Counter  cnt_type=Free Running  cnt_to=Inf  operation=Up  start_count=3  cnt_by_val=4  arith_type=Unsigned  n_bits=input_len_bits + 2  bin_pt=0  load_pin=off  rst=on  en=on  explicit_period=on  period=1  use_behavioral_HDL=off  implementation=Fabric  dbl_ovrd=off  block_type=counter
  we_delay1 : Subsystem  AncestorBlock=casper_library_delays/pipeline  mask(pipeline){latency=2}
      mask help:
      | An explicitly laid-out delay line to avoid mapping to SRL16s
      | for use in pipelining to help achieve timing closure.
      mask init:
      | pipeline_init(gcb,'latency',latency);
      settings: AttributesFormatString=Latency = %<latency>
      mask Display:
      | port_label('input', 1, 'd');
      | port_label('output', 1, 'q');
      | disp(['Z^-', num2str(latency)]);
  we_delay2 : Subsystem  AncestorBlock=casper_library_delays/pipeline  mask(pipeline){latency=2}
      mask help:
      | An explicitly laid-out delay line to avoid mapping to SRL16s
      | for use in pipelining to help achieve timing closure.
      mask init:
      | pipeline_init(gcb,'latency',latency);
      settings: AttributesFormatString=Latency = %<latency>
      mask Display:
      | port_label('input', 1, 'd');
      | port_label('output', 1, 'q');
      | disp(['Z^-', num2str(latency)]);
  we_delay3 : Subsystem  AncestorBlock=casper_library_delays/pipeline  mask(pipeline){latency=2}
      mask help:
      | An explicitly laid-out delay line to avoid mapping to SRL16s
      | for use in pipelining to help achieve timing closure.
      mask init:
      | pipeline_init(gcb,'latency',latency);
      settings: AttributesFormatString=Latency = %<latency>
      mask Display:
      | port_label('input', 1, 'd');
      | port_label('output', 1, 'q');
      | disp(['Z^-', num2str(latency)]);
  we_delay32 : Subsystem  AncestorBlock=casper_library_delays/pipeline  mask(pipeline){latency=2}
      mask help:
      | An explicitly laid-out delay line to avoid mapping to SRL16s
      | for use in pipelining to help achieve timing closure.
      mask init:
      | pipeline_init(gcb,'latency',latency);
      settings: AttributesFormatString=Latency = %<latency>
      mask Display:
      | port_label('input', 1, 'd');
      | port_label('output', 1, 'q');
      | disp(['Z^-', num2str(latency)]);
  we_delay4 : Subsystem  AncestorBlock=casper_library_delays/pipeline  mask(pipeline){latency=2}
      mask help:
      | An explicitly laid-out delay line to avoid mapping to SRL16s
      | for use in pipelining to help achieve timing closure.
      mask init:
      | pipeline_init(gcb,'latency',latency);
      settings: AttributesFormatString=Latency = %<latency>
      mask Display:
      | port_label('input', 1, 'd');
      | port_label('output', 1, 'q');
      | disp(['Z^-', num2str(latency)]);
  we_delay5 : Subsystem  AncestorBlock=casper_library_delays/pipeline  mask(pipeline){latency=2}
      mask help:
      | An explicitly laid-out delay line to avoid mapping to SRL16s
      | for use in pipelining to help achieve timing closure.
      mask init:
      | pipeline_init(gcb,'latency',latency);
      settings: AttributesFormatString=Latency = %<latency>
      mask Display:
      | port_label('input', 1, 'd');
      | port_label('output', 1, 'q');
      | disp(['Z^-', num2str(latency)]);
  we_delay6 : Subsystem  AncestorBlock=casper_library_delays/pipeline  mask(pipeline){latency=2}
      mask help:
      | An explicitly laid-out delay line to avoid mapping to SRL16s
      | for use in pipelining to help achieve timing closure.
      mask init:
      | pipeline_init(gcb,'latency',latency);
      settings: AttributesFormatString=Latency = %<latency>
      mask Display:
      | port_label('input', 1, 'd');
      | port_label('output', 1, 'q');
      | disp(['Z^-', num2str(latency)]);
  we_delay7 : Subsystem  AncestorBlock=casper_library_delays/pipeline  mask(pipeline){latency=2}
      mask help:
      | An explicitly laid-out delay line to avoid mapping to SRL16s
      | for use in pipelining to help achieve timing closure.
      mask init:
      | pipeline_init(gcb,'latency',latency);
      settings: AttributesFormatString=Latency = %<latency>
      mask Display:
      | port_label('input', 1, 'd');
      | port_label('output', 1, 'q');
      | disp(['Z^-', num2str(latency)]);
  d128 : Outport
  wires:
  dv/1 -> Assert1/1
  sync/1 -> Assert2/1
  p0_1/1 -> we_delay1/1(d)
  p0_2/1 -> we_delay2/1(d)
  p0_3/1 -> we_delay3/1(d)
  Concat20/1 -> Concat21/1, Concat21/2
  p0_0/1 -> we_delay32/1(d)
  Assert1/1 -> p0_0/2, Delay1/1, p0_3/2, p0_2/2, p0_1/2  "OUT_sync"
  Counter/1 -> Relational/2  "first_spec_ctr"
  Constant2/1 -> Relational/1
  Relational/1 -> Register/2
  Concat21/1 -> d128/1
  Register/1 -> Mux2/1, Logical/2  "first_spectrum"
  Logical/1 -> Counter/2
  Assert2/1 -> p0_0/1, Counter/1, Register/1, Register/3, p0_3/1, p0_2/1, p0_1/1
  Delay1/1 -> Logical/1
  we_delay32/1(q) -> convert_rd_en/1
  we_delay1/1(q) -> convert_rd_en1/1
  we_delay2/1(q) -> convert_rd_en2/1
  we_delay3/1(q) -> convert_rd_en3/1
  Mux2/1 -> Concat20/3, Concat20/5, Concat20/7, Concat20/1
  Constant10/1 -> Mux2/2
  Constant11/1 -> Mux2/3
  convert_rd_en/1 -> we_delay4/1(d)
  convert_rd_en1/1 -> we_delay5/1(d)
  convert_rd_en2/1 -> we_delay6/1(d)
  convert_rd_en3/1 -> we_delay7/1(d)
  we_delay4/1(q) -> Concat20/2
  we_delay5/1(q) -> Concat20/4
  we_delay6/1(q) -> Concat20/6
  we_delay7/1(q) -> Concat20/8
